simulink model "SMC_HighSidePwmDriver"  (R2021b)
settings: Solver=ode45  StartTime=0.0  StopTime=1  RelTol=1e-6  EnableMultiTasking=on
values from neighbouring files (symbols this model uses):
  C_s = tau_s/R_s    (= 0.1)    [SMC_HighSidePwmDriver_para.m]
  C_t = [c1 c2]    [SMC_HighSidePwmDriver_para.m]
  L = 0.1    [SMC_HighSidePwmDriver_para.m]
  R = 4    [SMC_HighSidePwmDriver_para.m]
  R_s = 0.1    [SMC_HighSidePwmDriver_para.m]
  T_R = [C_s*L 0; -L/R L]    [SMC_HighSidePwmDriver_para.m]
  T_s = 1/150    (= 0.00666666666667)    [SMC_HighSidePwmDriver_para.m]
  U_E = 12    [SMC_HighSidePwmDriver_para.m]
undefined symbols (not defined in the file or in its folder): C, DiscIntNeverNeededParam
libraries: spsSeriesRLCBranchLib x16, spsControlledCurrentSourceLib x4, spsCurrentMeasurementLib x4, spsDCVoltageSourceLib x4, spsDiodeLib x4, spsIdealSwitchLib x4, spsVoltageMeasurementLib x4, simulink x1, spspowerguiLib x1
settings Model: Creator=Hoffstadt  LastModifiedBy=w.schwamm
settings SolverCC: ZeroCrossControl=DisableAll  AlgebraicLoopSolver=TrustRegion
settings DataIOCC: LimitDataPoints=on  SaveFormat=Array  ReturnWorkspaceOutputs=off
settings OptimizationCC: LifeSpan=inf
settings DebuggingCC: UnderspecifiedInitializationDetection=Classic  MergeDetectMultiDrivingBlocksExec=none  SolverPrmCheckMsg=warning  StateNameClashWarn=warning  SFUnexpectedBacktrackingDiag=warning  SFNoUnconditionalDefaultTransitionDiag=warning  SFMachineParentedDataDiag=warning  ArithmeticOperatorsInVariantConditions=warning
settings HardwareCC: ProdBitPerPointer=32  ProdBitPerSizeT=32  ProdBitPerPtrDiffT=32  ProdLargestAtomicFloat=None  ProdIntDivRoundTo=Undefined  ProdEndianess=Unspecified  ProdWordSize=32  ProdHWDeviceType=32-bit Generic
settings ModelReferenceCC: PropagateSignalLabelsOutOfModel=off
settings SFSimCC: SimUseLocalCustomCode=off  CustomCodeUndefinedFunction=UseInterfaceOnly
settings RTWCC: RTWUseLocalCustomCode=off
settings CodeAppCC: StateflowObjectComments=on
settings GRTTargetCC: TargetLangStandard=C89/C90 (ANSI)
settings ConfigComp: CovMetricSettings=dw  CovSaveCumulativeToWorkspaceVar=on  CovSaveSingleToWorkspaceVar=on  CovExternalEMLEnable=off
settings SimscapeCC: SimscapeNormalizeSystem=off

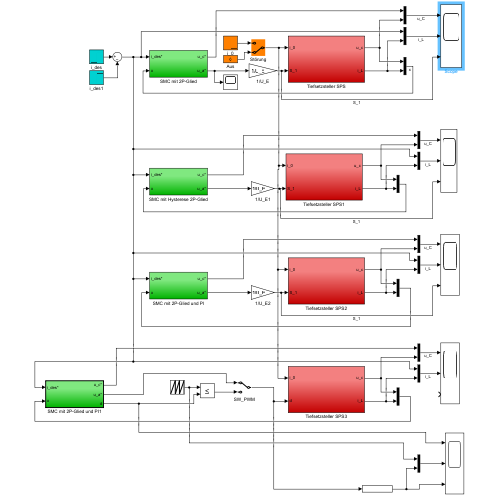
[thumbnail: Simulink's stored preview of the top-level diagram]
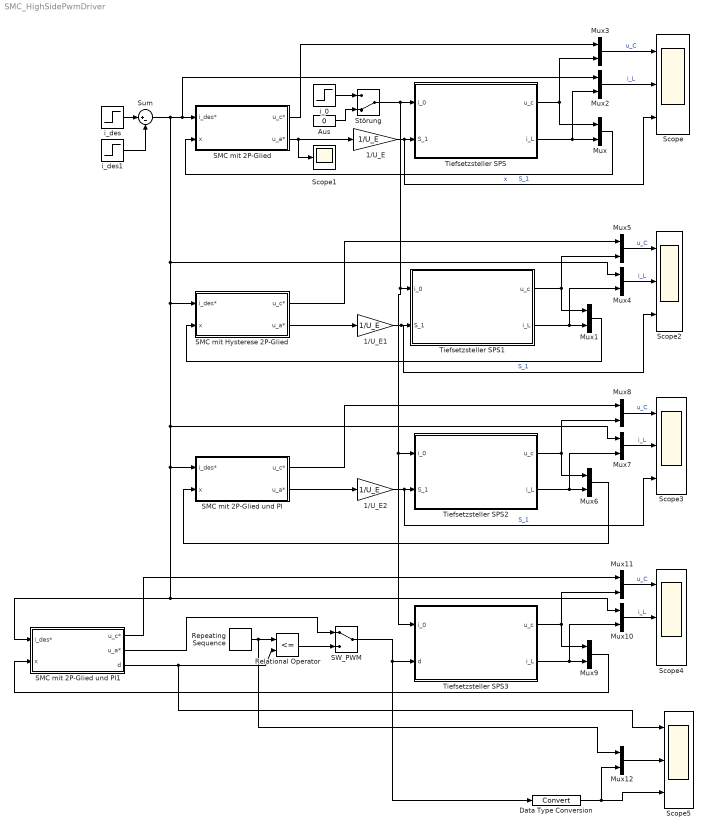
== system SMC_HighSidePwmDriver ==
  1/U_E : Gain  Gain=1/U_E
  1/U_E1 : Gain  Gain=1/U_E
  1/U_E2 : Gain  Gain=1/U_E
  Aus : Constant  Value=0
  Data Type Conversion : DataTypeConversion
  Mux{,1..12} (13 alike) : Mux  Inputs=2
  Relational Operator : RelationalOperator  Operator=<=  OutDataTypeStr=boolean  ZeroCross=off  RndMeth=Nearest
  Repeating Sequence : simulink/Sources/Repeating Sequence  rep_seq_t=[0 T_s]  rep_seq_y=[0 1]
  SMC mit 2P-Glied : Subsystem
  SMC mit 2P-Glied und PI : Subsystem
  SMC mit 2P-Glied und PI1 : Subsystem  TreatAsAtomicUnit=on  SystemSampleTime=0.001
  SMC mit Hysterese 2P-Glied : Subsystem
  SW_PWM : ManualSwitch
  Scope{,2..5} (5 alike) : Scope  NumInputPorts=3
  Scope1 : Scope
  Störung : ManualSwitch  CurrentSetting=0
  Sum : Sum  Inputs=|+-
  Tiefsetzsteller SPS : Subsystem
  Tiefsetzsteller SPS1 : Subsystem
  Tiefsetzsteller SPS2 : Subsystem
  Tiefsetzsteller SPS3 : Subsystem
  i_0 : Step  Time=150e-3  After=-0.5  SampleTime=0  ZeroCross=off
  i_des : Step  Time=0.05  After=1.0  SampleTime=0
  i_des1 : Step  Time=0.20  After=1.0  SampleTime=0
  wires:
  Tiefsetzsteller SPS/2(i_L) -> Mux2/2, Mux/2
  Tiefsetzsteller SPS/1(u_c) -> Mux3/2, Mux/1
  Mux2/1 -> Scope/2  "i_L"
  Mux3/1 -> Scope/1  "u_C"
  SMC mit 2P-Glied/2(u_a*) -> 1/U_E/1, Scope1/1
  Mux/1 -> SMC mit 2P-Glied/2(x)  "x"
  SMC mit 2P-Glied/1(u_c*) -> Mux3/1
  Aus/1 -> Störung/2
  i_0/1 -> Störung/1
  SMC mit Hysterese 2P-Glied/2(u_a*) -> 1/U_E1/1
  1/U_E/1 -> Scope/3, Tiefsetzsteller SPS/2(S_1)  "S_1"
  1/U_E1/1 -> Scope2/3, Tiefsetzsteller SPS1/2(S_1)  "S_1"
  Tiefsetzsteller SPS1/2(i_L) -> Mux4/2, Mux1/2
  Tiefsetzsteller SPS1/1(u_c) -> Mux1/1, Mux5/2
  Mux1/1 -> SMC mit Hysterese 2P-Glied/2(x)
  Mux4/1 -> Scope2/2  "i_L"
  Mux5/1 -> Scope2/1  "u_C"
  SMC mit Hysterese 2P-Glied/1(u_c*) -> Mux5/1
  SMC mit 2P-Glied und PI/2(u_a*) -> 1/U_E2/1
  1/U_E2/1 -> Scope3/3, Tiefsetzsteller SPS2/2(S_1)  "S_1"
  Tiefsetzsteller SPS2/2(i_L) -> Mux6/2, Mux7/2
  Tiefsetzsteller SPS2/1(u_c) -> Mux8/2, Mux6/1
  Mux6/1 -> SMC mit 2P-Glied und PI/2(x)
  Mux7/1 -> Scope3/2  "i_L"
  Mux8/1 -> Scope3/1  "u_C"
  SMC mit 2P-Glied und PI/1(u_c*) -> Mux8/1
  SMC mit 2P-Glied und PI1/1(u_c*) -> Mux11/1
  Mux11/1 -> Scope4/1  "u_C"
  Mux10/1 -> Scope4/2  "i_L"
  Mux9/1 -> SMC mit 2P-Glied und PI1/2(x)
  Tiefsetzsteller SPS3/1(u_c) -> Mux9/1, Mux11/2
  Tiefsetzsteller SPS3/2(i_L) -> Mux10/2, Mux9/2
  Störung/1 -> Tiefsetzsteller SPS3/1(i_0), Tiefsetzsteller SPS2/1(i_0), Tiefsetzsteller SPS1/1(i_0), Tiefsetzsteller SPS/1(i_0)
  Sum/1 -> SMC mit Hysterese 2P-Glied/1(i_des*), Mux7/1, Mux10/1, SMC mit 2P-Glied und PI1/1(i_des*), SMC mit 2P-Glied und PI/1(i_des*), Mux4/1, SMC mit 2P-Glied/1(i_des*), Mux2/1
  i_des/1 -> Sum/1
  i_des1/1 -> Sum/2
  Repeating Sequence/1 -> Relational Operator/1, Mux12/1
  SW_PWM/1 -> Data Type Conversion/1, Tiefsetzsteller SPS3/2(d)
  Data Type Conversion/1 -> Mux12/2, Scope5/3
  Relational Operator/1 -> SW_PWM/2
  SMC mit 2P-Glied und PI1/2(u_a*) -> SW_PWM/1
  SMC mit 2P-Glied und PI1/3(d) -> Scope5/1, Relational Operator/2
  Mux12/1 -> Scope5/2

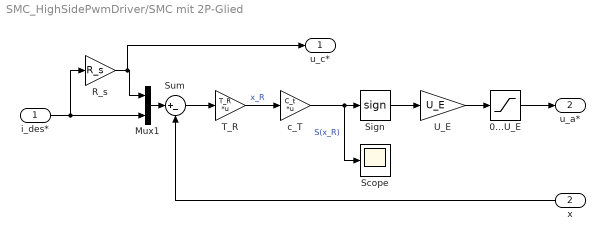
== system SMC_HighSidePwmDriver/SMC mit 2P-Glied ==
  i_des* : Inport
  x : Inport  Port=2
  0...U_E : Saturate  UpperLimit=U_E  LowerLimit=0  ZeroCross=off
  Mux1 : Mux  Inputs=2
  R_s : Gain  Gain=R_s
  Scope : Scope
  "Sign " : Signum  ZeroCross=off
  Sum : Sum  Inputs=|+-
  T_R : Gain  Gain=T_R  Multiplication=Matrix(K*u) (u vector)
  U_E : Gain  Gain=U_E
  c_T : Gain  Gain=C_t  Multiplication=Matrix(K*u) (u vector)
  u_c* : Outport
  u_a* : Outport  Port=2
  wires:
  x/1 -> Sum/2
  Mux1/1 -> Sum/1
  R_s/1 -> u_c*/1, Mux1/1
  i_des*/1 -> R_s/1, Mux1/2
  U_E/1 -> 0...U_E/1
  0...U_E/1 -> u_a*/1
  "Sign "/1 -> U_E/1
  c_T/1 -> Scope/1, "Sign "/1  "S(x_R)"
  T_R/1 -> c_T/1  "x_R"
  Sum/1 -> T_R/1

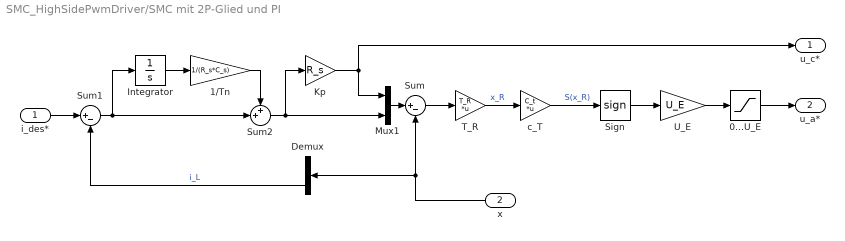
== system SMC_HighSidePwmDriver/SMC mit 2P-Glied und PI ==
  i_des* : Inport
  x : Inport  Port=2
  0...U_E : Saturate  UpperLimit=U_E  LowerLimit=0  ZeroCross=off
  1/Tn : Gain  Gain=1/(R_s*C_s)
  Demux : Demux  Outputs=2
  Integrator : Integrator
  Kp : Gain  Gain=R_s
  Mux1 : Mux  Inputs=2
  Sign : Signum  ZeroCross=off
  Sum : Sum  Inputs=|+-
  Sum1 : Sum  Inputs=|+-
  Sum2 : Sum  Inputs=++|
  T_R : Gain  Gain=T_R  Multiplication=Matrix(K*u) (u vector)
  U_E : Gain  Gain=U_E
  c_T : Gain  Gain=C_t  Multiplication=Matrix(K*u) (u vector)
  u_c* : Outport
  u_a* : Outport  Port=2
  wires:
  x/1 -> Demux/1, Sum/2
  Mux1/1 -> Sum/1
  Kp/1 -> u_c*/1, Mux1/1
  i_des*/1 -> Sum1/1
  U_E/1 -> 0...U_E/1
  0...U_E/1 -> u_a*/1
  Sign/1 -> U_E/1
  c_T/1 -> Sign/1  "S(x_R)"
  T_R/1 -> c_T/1  "x_R"
  Sum/1 -> T_R/1
  Sum2/1 -> Kp/1, Mux1/2
  1/Tn/1 -> Sum2/1
  Integrator/1 -> 1/Tn/1
  Sum1/1 -> Integrator/1, Sum2/2
  Demux/2 -> Sum1/2  "i_L"

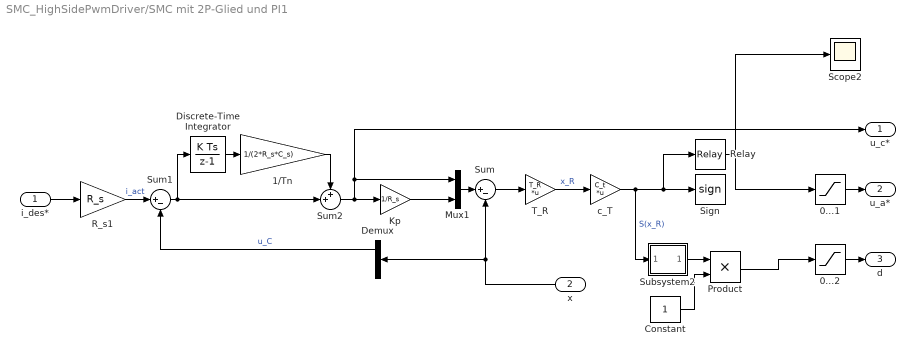
== system SMC_HighSidePwmDriver/SMC mit 2P-Glied und PI1 ==
  i_des* : Inport
  x : Inport  Port=2
  0...1 : Saturate  UpperLimit=1  LowerLimit=0  ZeroCross=off
  0...2 : Saturate  UpperLimit=1  LowerLimit=0  ZeroCross=off
  1/Tn : Gain  Gain=1/(2*R_s*C_s)
  Constant : Constant  SampleTime=-1
  Demux : Demux  Outputs=2
  Discrete-Time Integrator : DiscreteIntegrator  SampleTime=-1  ICPrevOutput=DiscIntNeverNeededParam  ICPrevScaledInput=DiscIntNeverNeededParam
  Kp : Gain  Gain=1/R_s
  Mux1 : Mux  Inputs=2
  Product : Product
  R_s1 : Gain  Gain=R_s
  Relay : Relay  OnSwitchValue=1e-3  OffSwitchValue=-1e-3  OffOutputValue=-1  ZeroCross=off
  Scope2 : Scope
  Sign : Signum  ZeroCross=off
  Subsystem2 : Subsystem  mask{delta=0.001}
      mask prompts: delta "Unit vector delta:"
      mask Display: disp('UnV')
  Sum : Sum  Inputs=|+-
  Sum1 : Sum  Inputs=|+-
  Sum2 : Sum  Inputs=++|
  T_R : Gain  Gain=T_R  Multiplication=Matrix(K*u) (u vector)
  c_T : Gain  Gain=C_t  Multiplication=Matrix(K*u) (u vector)
  u_c* : Outport
  u_a* : Outport  Port=2
  d : Outport  Port=3
  wires:
  Demux/1 -> Sum1/2  "u_C"
  Sum1/1 -> Discrete-Time Integrator/1, Sum2/2
  Discrete-Time Integrator/1 -> 1/Tn/1
  1/Tn/1 -> Sum2/1
  Sum/1 -> T_R/1
  T_R/1 -> c_T/1  "x_R"
  c_T/1 -> Relay/1, Sign/1, Subsystem2/1(In1)  "S(x_R)"
  i_des*/1 -> R_s1/1
  Mux1/1 -> Sum/1
  x/1 -> Sum/2, Demux/1
  0...1/1 -> u_a*/1
  Constant/1 -> Product/2
  Subsystem2/1(Out1) -> Product/1
  0...2/1 -> d/1
  Relay/1 -> 0...1/1, Scope2/1
  Product/1 -> 0...2/1
  R_s1/1 -> Sum1/1  "i_act"
  Kp/1 -> Mux1/2
  Sum2/1 -> u_c*/1, Mux1/1, Kp/1

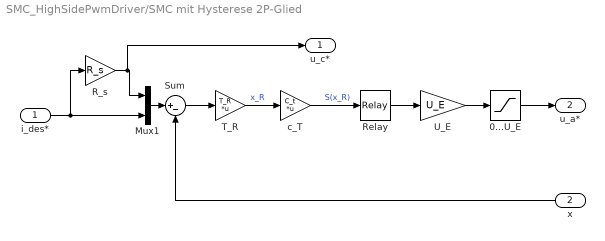
== system SMC_HighSidePwmDriver/SMC mit Hysterese 2P-Glied ==
  i_des* : Inport
  x : Inport  Port=2
  0...U_E : Saturate  UpperLimit=U_E  LowerLimit=0  ZeroCross=off
  Mux1 : Mux  Inputs=2
  R_s : Gain  Gain=R_s
  Relay : Relay  OnSwitchValue=1e-2  OffSwitchValue=-1e-2  OffOutputValue=-1  ZeroCross=off
  Sum : Sum  Inputs=|+-
  T_R : Gain  Gain=T_R  Multiplication=Matrix(K*u) (u vector)
  U_E : Gain  Gain=U_E
  c_T : Gain  Gain=C_t  Multiplication=Matrix(K*u) (u vector)
  u_c* : Outport
  u_a* : Outport  Port=2
  wires:
  Sum/1 -> T_R/1
  T_R/1 -> c_T/1  "x_R"
  Relay/1 -> U_E/1
  0...U_E/1 -> u_a*/1
  U_E/1 -> 0...U_E/1
  i_des*/1 -> Mux1/2, R_s/1
  R_s/1 -> Mux1/1, u_c*/1
  Mux1/1 -> Sum/1
  x/1 -> Sum/2
  c_T/1 -> Relay/1  "S(x_R)"

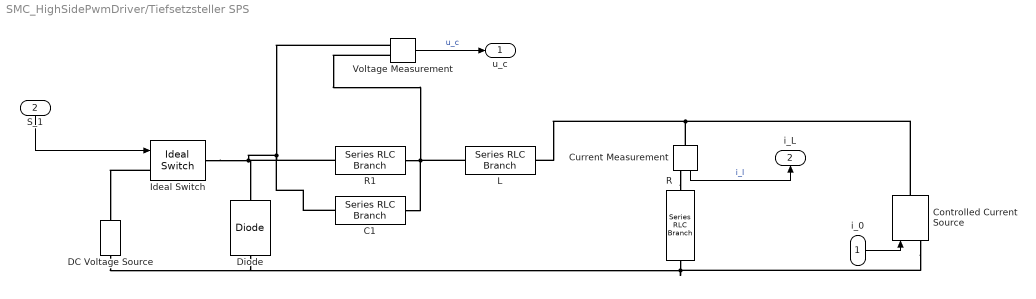
== system SMC_HighSidePwmDriver/Tiefsetzsteller SPS ==
  i_0 : Inport
  S_1 : Inport  Port=2
  C1 : spsSeriesRLCBranchLib/Series RLC Branch  LConnTagsString=__new0  RConnTagsString=__new0  BranchType=C  Resistance=R  Inductance=1e-3  SetiL0=off  InitialCurrent=0  Capacitance=C_s  Setx0=off  InitialVoltage=0  Measurements=None
  Controlled Current Source : spsControlledCurrentSourceLib/Controlled Current Source  Initialize=on  Source_Type=AC  Amplitude=0  Phase=0  Frequency=0  Measurements=None
  "Current Measurement " : spsCurrentMeasurementLib/Current Measurement  PhasorSimulation=off  OutputType=Complex  PSBequivalent=0
  DC Voltage Source : spsDCVoltageSourceLib/DC Voltage Source  Amplitude=U_E  Measurements=None
  "Diode " : spsDiodeLib/Diode  Ron=0.001  Lon=0  Vf=0  IC=0  UseSnubber=off  Rs=500  Cs=250e-9  Measurements=off
  "Ideal Switch " : spsIdealSwitchLib/Ideal Switch  Ron=0.001  Lon=0  IC=0  Rs=1e5  Cs=inf  Measurements=off
  L : spsSeriesRLCBranchLib/Series RLC Branch  LConnTagsString=__new0  RConnTagsString=__new0  BranchType=L  Resistance=R  Inductance=L  SetiL0=off  InitialCurrent=0  Capacitance=C  Setx0=off  InitialVoltage=0  Measurements=None
  R : spsSeriesRLCBranchLib/Series RLC Branch  LConnTagsString=__new0  RConnTagsString=__new0  BranchType=R  Resistance=R  Inductance=1e-3  SetiL0=off  InitialCurrent=0  Capacitance=1e-6  Setx0=off  InitialVoltage=0  Measurements=None
  R1 : spsSeriesRLCBranchLib/Series RLC Branch  LConnTagsString=__new0  RConnTagsString=__new0  BranchType=R  Resistance=R_s  Inductance=1e-3  SetiL0=off  InitialCurrent=0  Capacitance=1e-6  Setx0=off  InitialVoltage=0  Measurements=None
  Voltage Measurement : spsVoltageMeasurementLib/Voltage Measurement  PhasorSimulation=off  OutputType=Complex  PSBequivalent=0
  u_c : Outport
  i_L : Outport  Port=2
  wires:
  "Current Measurement "/1 -> i_L/1  "i_l"
  S_1/1 -> "Ideal Switch "/1
  i_0/1 -> Controlled Current Source/1
  Voltage Measurement/1 -> u_c/1  "u_c"
  connections:
  R/RConn1 -- DC Voltage Source/LConn1 -- "Diode "/LConn1 -- Controlled Current Source/LConn1
  "Ideal Switch "/RConn1 -- R1/LConn1 -- C1/LConn1 -- Voltage Measurement/LConn1 -- "Diode "/RConn1
  "Ideal Switch "/LConn1 -- DC Voltage Source/RConn1
  R1/RConn1 -- C1/RConn1 -- L/LConn1 -- Voltage Measurement/LConn2
  "Current Measurement "/RConn1 -- R/LConn1
  "Current Measurement "/LConn1 -- L/RConn1 -- Controlled Current Source/RConn1

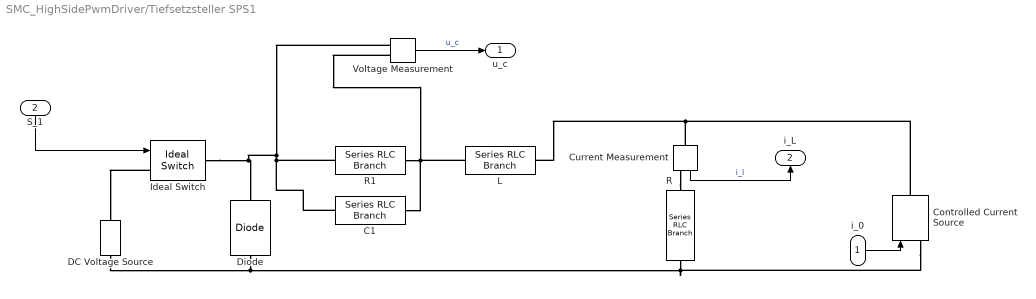
== system SMC_HighSidePwmDriver/Tiefsetzsteller SPS1 ==
  i_0 : Inport
  S_1 : Inport  Port=2
  C1 : spsSeriesRLCBranchLib/Series RLC Branch  LConnTagsString=__new0  RConnTagsString=__new0  BranchType=C  Resistance=R  Inductance=1e-3  SetiL0=off  InitialCurrent=0  Capacitance=C_s  Setx0=off  InitialVoltage=0  Measurements=None
  Controlled Current Source : spsControlledCurrentSourceLib/Controlled Current Source  Initialize=on  Source_Type=AC  Amplitude=0  Phase=0  Frequency=0  Measurements=None
  "Current Measurement " : spsCurrentMeasurementLib/Current Measurement  PhasorSimulation=off  OutputType=Complex  PSBequivalent=0
  DC Voltage Source : spsDCVoltageSourceLib/DC Voltage Source  Amplitude=U_E  Measurements=None
  "Diode " : spsDiodeLib/Diode  Ron=0.001  Lon=0  Vf=0  IC=0  UseSnubber=off  Rs=500  Cs=250e-9  Measurements=off
  "Ideal Switch " : spsIdealSwitchLib/Ideal Switch  Ron=0.001  Lon=0  IC=0  Rs=1e5  Cs=inf  Measurements=off
  L : spsSeriesRLCBranchLib/Series RLC Branch  LConnTagsString=__new0  RConnTagsString=__new0  BranchType=L  Resistance=R  Inductance=L  SetiL0=off  InitialCurrent=0  Capacitance=C  Setx0=off  InitialVoltage=0  Measurements=None
  R : spsSeriesRLCBranchLib/Series RLC Branch  LConnTagsString=__new0  RConnTagsString=__new0  BranchType=R  Resistance=R  Inductance=1e-3  SetiL0=off  InitialCurrent=0  Capacitance=1e-6  Setx0=off  InitialVoltage=0  Measurements=None
  R1 : spsSeriesRLCBranchLib/Series RLC Branch  LConnTagsString=__new0  RConnTagsString=__new0  BranchType=R  Resistance=R_s  Inductance=1e-3  SetiL0=off  InitialCurrent=0  Capacitance=1e-6  Setx0=off  InitialVoltage=0  Measurements=None
  Voltage Measurement : spsVoltageMeasurementLib/Voltage Measurement  PhasorSimulation=off  OutputType=Complex  PSBequivalent=0
  u_c : Outport
  i_L : Outport  Port=2
  wires:
  Voltage Measurement/1 -> u_c/1  "u_c"
  i_0/1 -> Controlled Current Source/1
  S_1/1 -> "Ideal Switch "/1
  "Current Measurement "/1 -> i_L/1  "i_l"
  connections:
  L/RConn1 -- "Current Measurement "/LConn1 -- Controlled Current Source/RConn1
  "Current Measurement "/RConn1 -- R/LConn1
  L/LConn1 -- R1/RConn1 -- Voltage Measurement/LConn2 -- C1/RConn1
  "Ideal Switch "/LConn1 -- DC Voltage Source/RConn1
  C1/LConn1 -- R1/LConn1 -- "Diode "/RConn1 -- "Ideal Switch "/RConn1 -- Voltage Measurement/LConn1
  Controlled Current Source/LConn1 -- "Diode "/LConn1 -- DC Voltage Source/LConn1 -- R/RConn1

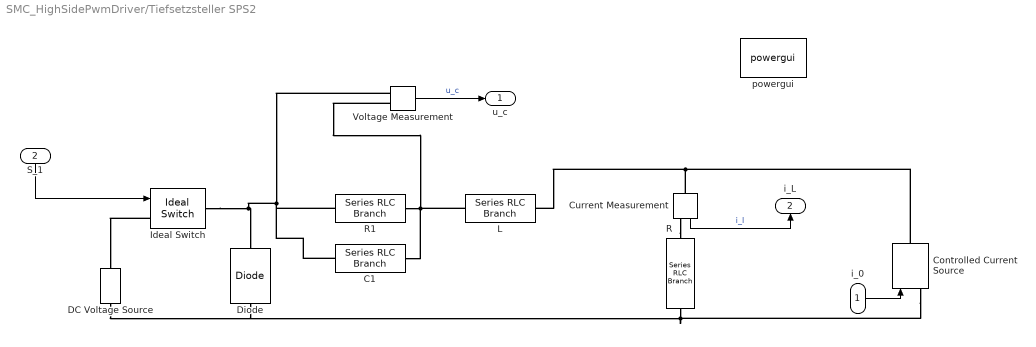
== system SMC_HighSidePwmDriver/Tiefsetzsteller SPS2 ==
  i_0 : Inport
  S_1 : Inport  Port=2
  C1 : spsSeriesRLCBranchLib/Series RLC Branch  LConnTagsString=__new0  RConnTagsString=__new0  BranchType=C  Resistance=R  Inductance=1e-3  SetiL0=off  InitialCurrent=0  Capacitance=C_s  Setx0=off  InitialVoltage=0  Measurements=None
  Controlled Current Source : spsControlledCurrentSourceLib/Controlled Current Source  Initialize=on  Source_Type=AC  Amplitude=0  Phase=0  Frequency=0  Measurements=None
  "Current Measurement " : spsCurrentMeasurementLib/Current Measurement  PhasorSimulation=off  OutputType=Complex  PSBequivalent=0
  DC Voltage Source : spsDCVoltageSourceLib/DC Voltage Source  Amplitude=U_E  Measurements=None
  "Diode " : spsDiodeLib/Diode  Ron=0.001  Lon=0  Vf=0  IC=0  UseSnubber=off  Rs=500  Cs=250e-9  Measurements=off
  "Ideal Switch " : spsIdealSwitchLib/Ideal Switch  Ron=0.001  Lon=0  IC=0  Rs=1e5  Cs=inf  Measurements=off
  L : spsSeriesRLCBranchLib/Series RLC Branch  LConnTagsString=__new0  RConnTagsString=__new0  BranchType=L  Resistance=R  Inductance=L  SetiL0=off  InitialCurrent=0  Capacitance=C  Setx0=off  InitialVoltage=0  Measurements=None
  R : spsSeriesRLCBranchLib/Series RLC Branch  LConnTagsString=__new0  RConnTagsString=__new0  BranchType=R  Resistance=R  Inductance=1e-3  SetiL0=off  InitialCurrent=0  Capacitance=1e-6  Setx0=off  InitialVoltage=0  Measurements=None
  R1 : spsSeriesRLCBranchLib/Series RLC Branch  LConnTagsString=__new0  RConnTagsString=__new0  BranchType=R  Resistance=R_s  Inductance=1e-3  SetiL0=off  InitialCurrent=0  Capacitance=1e-6  Setx0=off  InitialVoltage=0  Measurements=None
  Voltage Measurement : spsVoltageMeasurementLib/Voltage Measurement  PhasorSimulation=off  OutputType=Complex  PSBequivalent=0
  powergui : spspowerguiLib/powergui  Priority=1  SimulationMode=Continuous  SampleTime=50e-6  frequency=60  Iterations=50  frequencyindice=0  Pbase=100e6  ErrMax=1e-4  UnitsV=kV  UnitsW=MW  buscounter=0  FunctionMessages=off  echomessages=off  EnableUseOfTLC=off  CurrentSourceSwitches=on  DisableSnubberDevices=off  DisableRonSwitches=off  DisableVfSwitches=off  DisplayEquations=off  AutomaticDiscreteSolvers=off  SolverType=Tustin  Interpol=off  ExternalGateDelay=off  methode=off  Ts=0  x0status=blocks  SPID=off  SwTol=0  HookPort=off  NonlinearTolerance=1e-4  nMaxIteration=100  ContinueOnMaxIteration=off  RestoreLinks=warning  ResistiveCurrentMeasurement=off  Frange=[0:2:500]  Ylog=off  Xlog=on  ShowGrid=off  save=off  variable=ZData  structure=0  ZoomFFT=off  StartTime=0.0  cycles=1  DisplayStyle=1  fundamental=60  FreqAxis=off  MaxFrequency=1000  frequencyindicesteady=1  RmsSteady=1  display=off
  u_c : Outport
  i_L : Outport  Port=2
  wires:
  "Current Measurement "/1 -> i_L/1  "i_l"
  S_1/1 -> "Ideal Switch "/1
  i_0/1 -> Controlled Current Source/1
  Voltage Measurement/1 -> u_c/1  "u_c"
  connections:
  R/RConn1 -- DC Voltage Source/LConn1 -- "Diode "/LConn1 -- Controlled Current Source/LConn1
  Voltage Measurement/LConn1 -- "Ideal Switch "/RConn1 -- "Diode "/RConn1 -- R1/LConn1 -- C1/LConn1
  "Ideal Switch "/LConn1 -- DC Voltage Source/RConn1
  C1/RConn1 -- Voltage Measurement/LConn2 -- R1/RConn1 -- L/LConn1
  "Current Measurement "/RConn1 -- R/LConn1
  Controlled Current Source/RConn1 -- "Current Measurement "/LConn1 -- L/RConn1

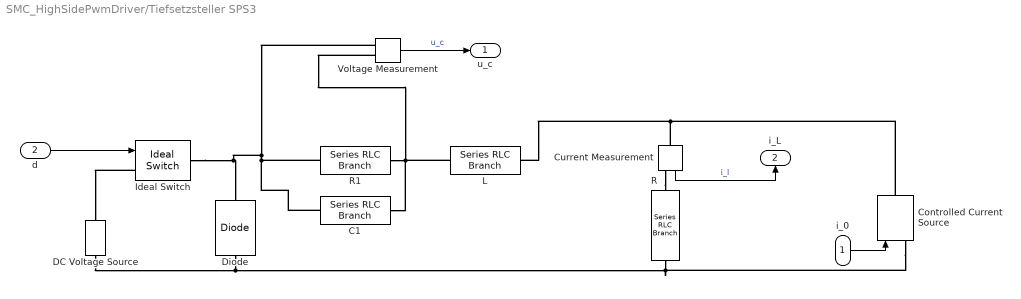
== system SMC_HighSidePwmDriver/Tiefsetzsteller SPS3 ==
  i_0 : Inport
  d : Inport  Port=2
  C1 : spsSeriesRLCBranchLib/Series RLC Branch  LConnTagsString=__new0  RConnTagsString=__new0  BranchType=C  Resistance=R  Inductance=1e-3  SetiL0=off  InitialCurrent=0  Capacitance=C_s  Setx0=off  InitialVoltage=0  Measurements=None
  Controlled Current Source : spsControlledCurrentSourceLib/Controlled Current Source  Initialize=on  Source_Type=AC  Amplitude=0  Phase=0  Frequency=0  Measurements=None
  "Current Measurement " : spsCurrentMeasurementLib/Current Measurement  PhasorSimulation=off  OutputType=Complex  PSBequivalent=0
  DC Voltage Source : spsDCVoltageSourceLib/DC Voltage Source  Amplitude=U_E  Measurements=None
  "Diode " : spsDiodeLib/Diode  Ron=0.001  Lon=0  Vf=0  IC=0  UseSnubber=off  Rs=500  Cs=250e-9  Measurements=off
  "Ideal Switch " : spsIdealSwitchLib/Ideal Switch  Ron=0.001  Lon=0  IC=0  Rs=1e5  Cs=inf  Measurements=off
  L : spsSeriesRLCBranchLib/Series RLC Branch  LConnTagsString=__new0  RConnTagsString=__new0  BranchType=L  Resistance=R  Inductance=L  SetiL0=off  InitialCurrent=0  Capacitance=C  Setx0=off  InitialVoltage=0  Measurements=None
  R : spsSeriesRLCBranchLib/Series RLC Branch  LConnTagsString=__new0  RConnTagsString=__new0  BranchType=R  Resistance=1*R  Inductance=1e-3  SetiL0=off  InitialCurrent=0  Capacitance=1e-6  Setx0=off  InitialVoltage=0  Measurements=None
  R1 : spsSeriesRLCBranchLib/Series RLC Branch  LConnTagsString=__new0  RConnTagsString=__new0  BranchType=R  Resistance=R_s  Inductance=1e-3  SetiL0=off  InitialCurrent=0  Capacitance=1e-6  Setx0=off  InitialVoltage=0  Measurements=None
  Voltage Measurement : spsVoltageMeasurementLib/Voltage Measurement  PhasorSimulation=off  OutputType=Complex  PSBequivalent=0
  u_c : Outport
  i_L : Outport  Port=2
  wires:
  Voltage Measurement/1 -> u_c/1  "u_c"
  i_0/1 -> Controlled Current Source/1
  "Current Measurement "/1 -> i_L/1  "i_l"
  d/1 -> "Ideal Switch "/1
  connections:
  L/RConn1 -- "Current Measurement "/LConn1 -- Controlled Current Source/RConn1
  "Current Measurement "/RConn1 -- R/LConn1
  L/LConn1 -- R1/RConn1 -- Voltage Measurement/LConn2 -- C1/RConn1
  "Ideal Switch "/LConn1 -- DC Voltage Source/RConn1
  C1/LConn1 -- R1/LConn1 -- "Diode "/RConn1 -- "Ideal Switch "/RConn1 -- Voltage Measurement/LConn1
  Controlled Current Source/LConn1 -- "Diode "/LConn1 -- DC Voltage Source/LConn1 -- R/RConn1

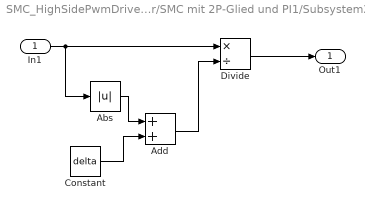
== system SMC_HighSidePwmDriver/SMC mit 2P-Glied und PI1/Subsystem2 ==
  In1 : Inport
  Abs : Abs  ZeroCross=off
  Add : Sum
  Constant : Constant  Value=delta  SampleTime=-1
  Divide : Product  Inputs=*/
  Out1 : Outport
  wires:
  In1/1 -> Abs/1, Divide/1
  Divide/1 -> Out1/1
  Abs/1 -> Add/1
  Add/1 -> Divide/2
  Constant/1 -> Add/2
